simulink model "SF015A_WhlImbRejctn"  (R2013b)
settings: Solver=FixedStepDiscrete  SolverMode=SingleTasking  StartTime=0.0  StopTime=1  FixedStep=0.002  RelTol=1e-3
values from neighbouring files (symbols this model uses):
  ACTIVBANDMAX_ULS_U32 = DataDict.Constant    [SF015A_WhlImbRejctn_DataDict.m]
  ADAPVFILMAX_ULS_F32 = DataDict.Constant    [SF015A_WhlImbRejctn_DataDict.m]
  ARCHGLBPRM_180OVERPI_ULS_F32 = DataDict.Constant    [SF015A_WhlImbRejctn_DataDict.m]
  ARCHGLBPRM_2MILLISEC_SEC_F32 = DataDict.Constant    [SF015A_WhlImbRejctn_DataDict.m]
  ARCHGLBPRM_2PI_ULS_F32 = DataDict.Constant    [SF015A_WhlImbRejctn_DataDict.m]
  ARCHGLBPRM_FLOATZEROTHD_ULS_F32 = DataDict.Constant    [SF015A_WhlImbRejctn_DataDict.m]
  ARCHGLBPRM_PI_ULS_F32 = DataDict.Constant    [SF015A_WhlImbRejctn_DataDict.m]
  ARCHGLBPRM_PIOVER180_ULS_F32 = DataDict.Constant    [SF015A_WhlImbRejctn_DataDict.m]
  ARCHGLBPRM_PIOVER2_ULS_F32 = DataDict.Constant    [SF015A_WhlImbRejctn_DataDict.m]
  CALMINSPERCOUNT_ULS_F32 = DataDict.Constant    [SF015A_WhlImbRejctn_DataDict.m]
  DURATIONDISABLE_CNT_U16 = DataDict.Constant    [SF015A_WhlImbRejctn_DataDict.m]
  FILTWHLSPDMAX_MOTRADPERSEC_F32 = DataDict.Constant    [SF015A_WhlImbRejctn_DataDict.m]
  MICROSECTOMILLISEC_ULS_F32 = DataDict.Constant    [SF015A_WhlImbRejctn_DataDict.m]
  MINSTOMILLISEC_ULS_F32 = DataDict.Constant    [SF015A_WhlImbRejctn_DataDict.m]
  NINETY_ULS_F32 = DataDict.Constant    [SF015A_WhlImbRejctn_DataDict.m]
  NODEBSTEP_CNT_U16 = DataDict.Constant    [SF015A_WhlImbRejctn_DataDict.m]
  NROFDLY_CNT_U08 = DataDict.Constant    [SF015A_WhlImbRejctn_DataDict.m]
  ONEHALF_ULS_F32 = DataDict.Constant    [SF015A_WhlImbRejctn_DataDict.m]
  ONEHUNDRED_ULS_F32 = DataDict.Constant    [SF015A_WhlImbRejctn_DataDict.m]
  ONEOVRTHREE_ULS_F32 = DataDict.Constant    [SF015A_WhlImbRejctn_DataDict.m]
  ONEOVRTWENTY_ULS_F32 = DataDict.Constant    [SF015A_WhlImbRejctn_DataDict.m]
  ONETHOUSAND_ULS_F32 = DataDict.Constant    [SF015A_WhlImbRejctn_DataDict.m]
  PEAKMAX_ULS_F32 = DataDict.Constant    [SF015A_WhlImbRejctn_DataDict.m]
  PEAKMIN_ULS_F32 = DataDict.Constant    [SF015A_WhlImbRejctn_DataDict.m]
  PHAADJMAX_ULS_F32 = DataDict.Constant    [SF015A_WhlImbRejctn_DataDict.m]
  PITIMESSAMPLETIME_ULS_F32 = DataDict.Constant    [SF015A_WhlImbRejctn_DataDict.m]
  STOREDMINSPERCOUNT_ULS_F32 = DataDict.Constant    [SF015A_WhlImbRejctn_DataDict.m]
  TWO_ULS_F32 = DataDict.Constant    [SF015A_WhlImbRejctn_DataDict.m]
  TWOOVRTHREE_ULS_F32 = DataDict.Constant    [SF015A_WhlImbRejctn_DataDict.m]
  WhlImbRejctnAdpvFac = DataDict.Calibration    [SF015A_WhlImbRejctn_DataDict.m]
  WhlImbRejctnAutScaEna = DataDict.Calibration    [SF015A_WhlImbRejctn_DataDict.m]
  WhlImbRejctnAutScaTar = DataDict.Calibration    [SF015A_WhlImbRejctn_DataDict.m]
  WhlImbRejctnCurrMgnSlewPerLoop = DataDict.Calibration    [SF015A_WhlImbRejctn_DataDict.m]
  WhlImbRejctnDcTrendFltRcvryDly = DataDict.Calibration    [SF015A_WhlImbRejctn_DataDict.m]
  WhlImbRejctnDcTrendFltRcvryNegStep = DataDict.Calibration    [SF015A_WhlImbRejctn_DataDict.m]
  WhlImbRejctnDcTrendFltRcvryPosStep = DataDict.Calibration    [SF015A_WhlImbRejctn_DataDict.m]
  WhlImbRejctnDcTrendFltRcvryThd = DataDict.Calibration    [SF015A_WhlImbRejctn_DataDict.m]
  WhlImbRejctnDcTrendTh2Tq = DataDict.Calibration    [SF015A_WhlImbRejctn_DataDict.m]
  WhlImbRejctnDcTrendThTq = DataDict.Calibration    [SF015A_WhlImbRejctn_DataDict.m]
  WhlImbRejctnDcTrendTi2Sec = DataDict.Calibration    [SF015A_WhlImbRejctn_DataDict.m]
  WhlImbRejctnDcTrendTiSec = DataDict.Calibration    [SF015A_WhlImbRejctn_DataDict.m]
  WhlImbRejctnEnaSlewPerLoop = DataDict.Calibration    [SF015A_WhlImbRejctn_DataDict.m]
  WhlImbRejctnFctEna = DataDict.Calibration    [SF015A_WhlImbRejctn_DataDict.m]
  WhlImbRejctnFrqDiagcAmpThd = DataDict.Calibration    [SF015A_WhlImbRejctn_DataDict.m]
  WhlImbRejctnFrqDiagcEna = DataDict.Calibration    [SF015A_WhlImbRejctn_DataDict.m]
  WhlImbRejctnFrqDiagcFltRcvryDly = DataDict.Calibration    [SF015A_WhlImbRejctn_DataDict.m]
  WhlImbRejctnFrqDiagcFltRcvryNegStep = DataDict.Calibration    [SF015A_WhlImbRejctn_DataDict.m]
  WhlImbRejctnFrqDiagcFltRcvryPosStep = DataDict.Calibration    [SF015A_WhlImbRejctn_DataDict.m]
  WhlImbRejctnFrqDiagcFltRcvryThd = DataDict.Calibration    [SF015A_WhlImbRejctn_DataDict.m]
  WhlImbRejctnFrqDiagcThd = DataDict.Calibration    [SF015A_WhlImbRejctn_DataDict.m]
  WhlImbRejctnFrqDiagcTout = DataDict.Calibration    [SF015A_WhlImbRejctn_DataDict.m]
  WhlImbRejctnFrqDiagcUgrPoleMgn = DataDict.Calibration    [SF015A_WhlImbRejctn_DataDict.m]
  WhlImbRejctnFrqScaTblX = DataDict.Calibration    [SF015A_WhlImbRejctn_DataDict.m]
  WhlImbRejctnMaxDurn = DataDict.Calibration    [SF015A_WhlImbRejctn_DataDict.m]
  WhlImbRejctnMaxMgn = DataDict.Calibration    [SF015A_WhlImbRejctn_DataDict.m]
  WhlImbRejctnMaxMgnFltNegStep = DataDict.Calibration    [SF015A_WhlImbRejctn_DataDict.m]
  WhlImbRejctnMaxMgnFltPosStep = DataDict.Calibration    [SF015A_WhlImbRejctn_DataDict.m]
  WhlImbRejctnMaxMgnFltRcvryDly = DataDict.Calibration    [SF015A_WhlImbRejctn_DataDict.m]
  WhlImbRejctnMaxMgnFltRcvryNegStep = DataDict.Calibration    [SF015A_WhlImbRejctn_DataDict.m]
  WhlImbRejctnMaxMgnFltRcvryPosStep = DataDict.Calibration    [SF015A_WhlImbRejctn_DataDict.m]
  WhlImbRejctnMaxMgnFltRcvryThd = DataDict.Calibration    [SF015A_WhlImbRejctn_DataDict.m]
  WhlImbRejctnMaxMgnFltThd = DataDict.Calibration    [SF015A_WhlImbRejctn_DataDict.m]
  WhlImbRejctnMgnEstimnDeltaSca = DataDict.Calibration    [SF015A_WhlImbRejctn_DataDict.m]
  WhlImbRejctnMgnEstimnDiThd = DataDict.Calibration    [SF015A_WhlImbRejctn_DataDict.m]
  WhlImbRejctnMgnEstimnEnaThd = DataDict.Calibration    [SF015A_WhlImbRejctn_DataDict.m]
  WhlImbRejctnMgnEstimnFrq = DataDict.Calibration    [SF015A_WhlImbRejctn_DataDict.m]
  WhlImbRejctnMgnEstimnFrqDelta = DataDict.Calibration    [SF015A_WhlImbRejctn_DataDict.m]
  WhlImbRejctnMgnEstimnLeak = DataDict.Calibration    [SF015A_WhlImbRejctn_DataDict.m]
  WhlImbRejctnRampDwnTi = DataDict.Calibration    [SF015A_WhlImbRejctn_DataDict.m]
  WhlImbRejctnScaCncl = DataDict.Calibration    [SF015A_WhlImbRejctn_DataDict.m]
  WhlImbRejctnUgrPoleMgn = DataDict.Calibration    [SF015A_WhlImbRejctn_DataDict.m]
  WhlImbRejctnVehSpdEna = DataDict.Calibration    [SF015A_WhlImbRejctn_DataDict.m]
  WhlImbRejctnWhlSpdCorrlnFltRcvryDly = DataDict.Calibration    [SF015A_WhlImbRejctn_DataDict.m]
  WhlImbRejctnWhlSpdCorrlnFltRcvryNegStep = DataDict.Calibration    [SF015A_WhlImbRejctn_DataDict.m]
  WhlImbRejctnWhlSpdCorrlnFltRcvryPosStep = DataDict.Calibration    [SF015A_WhlImbRejctn_DataDict.m]
  WhlImbRejctnWhlSpdCorrlnFltRcvryThd = DataDict.Calibration    [SF015A_WhlImbRejctn_DataDict.m]
  WhlImbRejctnWhlSpdCorrlnThd = DataDict.Calibration    [SF015A_WhlImbRejctn_DataDict.m]
  WhlImbRejctnWhlSpdCorrlnTi = DataDict.Calibration    [SF015A_WhlImbRejctn_DataDict.m]
  WIRCMDMAX_MOTNWTMTR_F32 = DataDict.Constant    [SF015A_WhlImbRejctn_DataDict.m]
  ZERO_ULS_F32 = DataDict.Constant    [SF015A_WhlImbRejctn_DataDict.m]
undefined symbols (not defined in the file or in its folder): Cntr, NtcNr1, NvmGetErrSts1, SigQlfr1, Sts, SysSt1
libraries: simulink x32, FixdToFloat x32, Fil x20, NxtrLim x15, NxtrNvM x12, NxtrAbslt x8, NxtrMath x7, NxtrMax x6, NxtrMin x4, FloatToFixd x2, LnrIntrpn x2, NxtrSign x1
(part 5 of 12)

== system SF015A_WhlImbRejctn/WhlImbRejctn/WhlImbRejctnPer2/Flt Recovery- DC Trend/Update Fault Status ==
  Structvar : Inport
  Status : Inport  Port=2
  Bus Assignment : BusAssignment  AssignedSignals=Cntr,Sts
  Bus Selector : BusSelector  OutputSignals=Cntr,Sts,Thd,NegStep,PosStep
  Compare To Zero : simulink/Logic and Bit Operations/Compare To Zero  relop=<=  OutDataTypeStr=boolean
  Constant : Constant  Value=0  OutDataTypeStr=single
  CopyRight2 : Subsystem  Description=|  mask(Copyright Information){none=on}
      | Copyright info block.                                               
      |                                                                     
      | Place copyright information at the top of every subsystem in design.
      mask prompts: none "No parameters"
      mask help: Place copyright information at the top of every subsystem in design.
      mask Display:
      | NxtrConf = 'Nexteer Confidential';
      | 
      | sys = bdroot; %handle for the current model ("system")
      | first = get_param(sys,'Created');
      | first = first(end-3:end);  %year is last four digits
      | 
      | last = get_param(sys,'LastModifiedDate');
      | if isempty(last)
      |     last = datestr(now,'yyyy');
      | else
      |     last = last(end-3:end);
      | end
      | 
      | if strcmp(first,last)
      |     fprintf('%s -- Copyright %s Nexteer',NxtrConf,first)
      | else
      |     fprintf('%s -- %s%s- %s Nexteer',NxtrConf,char(169),first,last)
      | end
  Enumerated Constant : simulink/Sources/Enumerated Constant  OutDataTypeStr=Enum: SigQlfr1  Value=SigQlfr1.SIGQLFR_FAILD  SampleTime=inf
  Enumerated Constant1 : simulink/Sources/Enumerated Constant  OutDataTypeStr=Enum: SigQlfr1  Value=SigQlfr1.SIGQLFR_PASSD  SampleTime=inf
  If : If  IfExpression=u1
  If1 : If  NumInputs=2  IfExpression=u1  ElseIfExpressions=u2  ShowElse=off
  Merge : Merge
  Relational Operator : RelationalOperator  OutDataTypeStr=boolean
  Terminator : Terminator
  Towards Failed : Subsystem  TreatAsAtomicUnit=on
  Towards Passed : Subsystem  TreatAsAtomicUnit=on
  Update to Failed : Subsystem  TreatAsAtomicUnit=on
  Update to Passed : Subsystem  TreatAsAtomicUnit=on
  counter : Merge
  Structvar_out : Outport
  wires:
  Structvar/1 -> Bus Assignment/1, Bus Selector/1
  Status/1 -> If/1
  If/1 -> Towards Failed/Action
  If/2 -> Towards Passed/Action
  [PosStep] -> Towards Failed/1(PosStep)
  [NegStep] -> Towards Passed/1(NegStep)
  Towards Failed/1(Out1) -> counter/1
  Towards Passed/1(Out1) -> counter/2
  [Cnt] -> Towards Failed/2(Cnt)
  [Thd] -> Towards Failed/3(Thd)
  Constant/1 -> Towards Passed/3(Thd)
  counter/1 -> [Cnt_update], Compare To Zero/1, Relational Operator/1
  Relational Operator/1 -> If1/1
  If1/1 -> Update to Failed/Action
  If1/2 -> Update to Passed/Action
  Compare To Zero/1 -> If1/2
  Enumerated Constant1/1 -> Update to Passed/1(In1)
  Update to Failed/1(Out1) -> Merge/1
  Update to Passed/1(Out1) -> Merge/2
  Enumerated Constant/1 -> Update to Failed/1(In1)
  Bus Assignment/1 -> Structvar_out/1
  Merge/1 -> [Sts_update]
  Bus Selector/1 -> [Cnt]  "<Cntr>"
  Bus Selector/3 -> [Thd]  "<Thd>"
  Bus Selector/4 -> [NegStep]  "<NegStep>"
  Bus Selector/5 -> [PosStep]  "<PosStep>"
  [Cnt_update] -> Bus Assignment/2
  [Sts_update] -> Bus Assignment/3
  [Cnt] -> Towards Passed/2(Cnt)
  [Thd] -> Relational Operator/2
  Bus Selector/2 -> Terminator/1  "<Sts>"

== system SF015A_WhlImbRejctn/WhlImbRejctn/WhlImbRejctnPer2/Flt Recovery- Freq Diag/CopyRight2 ==

== system SF015A_WhlImbRejctn/WhlImbRejctn/WhlImbRejctnPer2/Flt Recovery- Freq Diag/ElapsedTime1 ==
  FltStsTrue : Inport
  CopyRight2 : Subsystem  Description=|  mask(Copyright Information){none=on}
      | Copyright info block.                                               
      |                                                                     
      | Place copyright information at the top of every subsystem in design.
      mask prompts: none "No parameters"
      mask help: Place copyright information at the top of every subsystem in design.
      mask Display:
      | NxtrConf = 'Nexteer Confidential';
      | 
      | sys = bdroot; %handle for the current model ("system")
      | first = get_param(sys,'Created');
      | first = first(end-3:end);  %year is last four digits
      | 
      | last = get_param(sys,'LastModifiedDate');
      | if isempty(last)
      |     last = datestr(now,'yyyy');
      | else
      |     last = last(end-3:end);
      | end
      | 
      | if strcmp(first,last)
      |     fprintf('%s -- Copyright %s Nexteer',NxtrConf,first)
      | else
      |     fprintf('%s -- %s%s- %s Nexteer',NxtrConf,char(169),first,last)
      | end
  Data Store Read : DataStoreRead  Priority=1  DataStoreName=FrqDiagcLrngEnaPrev
      settings: AttributesFormatString="priority:  %<Priority>"
  Data Store Write : DataStoreWrite  Priority=2  DataStoreName=FrqDiagcLrngEnaPrev
      settings: AttributesFormatString="priority:  %<Priority>"
  If : If  NumInputs=2  IfExpression=u1  ElseIfExpressions=u2
  If not true elapsed time = 0 : Subsystem  TreatAsAtomicUnit=on
  "If true and last step is true calculate elapsed time " : Subsystem  TreatAsAtomicUnit=on
  "If true and last step not true elapsed time = 0 get reference time " : Subsystem  TreatAsAtomicUnit=on
  Logical Operator1 : Logic  Operator=NOT  AllPortsSameDT=off  OutDataTypeStr=boolean
  Logical Operator2 : Logic  Operator=NOT  AllPortsSameDT=off  OutDataTypeStr=boolean
  Merge : Merge  Inputs=3
  ElapsedTime : Outport
  wires:
  If/1 -> If not true elapsed time = 0/Action
  If/2 -> "If true and last step not true elapsed time = 0 get reference time "/Action
  If/3 -> "If true and last step is true calculate elapsed time "/Action
  If not true elapsed time = 0/1(SpanTi) -> Merge/1
  "If true and last step not true elapsed time = 0 get reference time "/1("SpanTi ") -> Merge/2
  "If true and last step is true calculate elapsed time "/1(SpanTi) -> Merge/3
  Merge/1 -> ElapsedTime/1
  FltStsTrue/1 -> Logical Operator2/1, Data Store Write/1
  Data Store Read/1 -> Logical Operator1/1
  Logical Operator2/1 -> If/1
  Logical Operator1/1 -> If/2

== system SF015A_WhlImbRejctn/WhlImbRejctn/WhlImbRejctnPer2/Flt Recovery- Freq Diag/Update Fault Status ==
  Structvar : Inport
  Status : Inport  Port=2
  Bus Assignment : BusAssignment  AssignedSignals=Cntr,Sts
  Bus Selector : BusSelector  OutputSignals=Cntr,Sts,Thd,NegStep,PosStep
  Compare To Zero : simulink/Logic and Bit Operations/Compare To Zero  relop=<=  OutDataTypeStr=boolean
  Constant : Constant  Value=0  OutDataTypeStr=single
  CopyRight2 : Subsystem  Description=|  mask(Copyright Information){none=on}
      | Copyright info block.                                               
      |                                                                     
      | Place copyright information at the top of every subsystem in design.
      mask prompts: none "No parameters"
      mask help: Place copyright information at the top of every subsystem in design.
      mask Display:
      | NxtrConf = 'Nexteer Confidential';
      | 
      | sys = bdroot; %handle for the current model ("system")
      | first = get_param(sys,'Created');
      | first = first(end-3:end);  %year is last four digits
      | 
      | last = get_param(sys,'LastModifiedDate');
      | if isempty(last)
      |     last = datestr(now,'yyyy');
      | else
      |     last = last(end-3:end);
      | end
      | 
      | if strcmp(first,last)
      |     fprintf('%s -- Copyright %s Nexteer',NxtrConf,first)
      | else
      |     fprintf('%s -- %s%s- %s Nexteer',NxtrConf,char(169),first,last)
      | end
  Enumerated Constant : simulink/Sources/Enumerated Constant  OutDataTypeStr=Enum: SigQlfr1  Value=SigQlfr1.SIGQLFR_FAILD  SampleTime=inf
  Enumerated Constant1 : simulink/Sources/Enumerated Constant  OutDataTypeStr=Enum: SigQlfr1  Value=SigQlfr1.SIGQLFR_PASSD  SampleTime=inf
  If : If  IfExpression=u1
  If1 : If  NumInputs=2  IfExpression=u1  ElseIfExpressions=u2  ShowElse=off
  Merge : Merge
  Relational Operator : RelationalOperator  OutDataTypeStr=boolean
  Terminator : Terminator
  Towards Failed : Subsystem  TreatAsAtomicUnit=on
  Towards Passed : Subsystem  TreatAsAtomicUnit=on
  Update to Failed : Subsystem  TreatAsAtomicUnit=on
  Update to Passed : Subsystem  TreatAsAtomicUnit=on
  counter : Merge
  Structvar_out : Outport
  wires:
  Structvar/1 -> Bus Assignment/1, Bus Selector/1
  Status/1 -> If/1
  If/1 -> Towards Failed/Action
  If/2 -> Towards Passed/Action
  [PosStep] -> Towards Failed/1(PosStep)
  [NegStep] -> Towards Passed/1(NegStep)
  Towards Failed/1(Out1) -> counter/1
  Towards Passed/1(Out1) -> counter/2
  [Cnt] -> Towards Failed/2(Cnt)
  [Thd] -> Towards Failed/3(Thd)
  Constant/1 -> Towards Passed/3(Thd)
  counter/1 -> [Cnt_update], Compare To Zero/1, Relational Operator/1
  Relational Operator/1 -> If1/1
  If1/1 -> Update to Failed/Action
  If1/2 -> Update to Passed/Action
  Compare To Zero/1 -> If1/2
  Enumerated Constant1/1 -> Update to Passed/1(In1)
  Update to Failed/1(Out1) -> Merge/1
  Update to Passed/1(Out1) -> Merge/2
  Enumerated Constant/1 -> Update to Failed/1(In1)
  Bus Assignment/1 -> Structvar_out/1
  Merge/1 -> [Sts_update]
  Bus Selector/1 -> [Cnt]  "<Cntr>"
  Bus Selector/3 -> [Thd]  "<Thd>"
  Bus Selector/4 -> [NegStep]  "<NegStep>"
  Bus Selector/5 -> [PosStep]  "<PosStep>"
  [Cnt_update] -> Bus Assignment/2
  [Sts_update] -> Bus Assignment/3
  [Cnt] -> Towards Passed/2(Cnt)
  [Thd] -> Relational Operator/2
  Bus Selector/2 -> Terminator/1  "<Sts>"

== system SF015A_WhlImbRejctn/WhlImbRejctn/WhlImbRejctnPer2/Flt Recovery- Max Mag/CopyRight2 ==

== system SF015A_WhlImbRejctn/WhlImbRejctn/WhlImbRejctnPer2/Flt Recovery- Max Mag/ElapsedTime1 ==
  FltStsTrue : Inport
  CopyRight2 : Subsystem  Description=|  mask(Copyright Information){none=on}
      | Copyright info block.                                               
      |                                                                     
      | Place copyright information at the top of every subsystem in design.
      mask prompts: none "No parameters"
      mask help: Place copyright information at the top of every subsystem in design.
      mask Display:
      | NxtrConf = 'Nexteer Confidential';
      | 
      | sys = bdroot; %handle for the current model ("system")
      | first = get_param(sys,'Created');
      | first = first(end-3:end);  %year is last four digits
      | 
      | last = get_param(sys,'LastModifiedDate');
      | if isempty(last)
      |     last = datestr(now,'yyyy');
      | else
      |     last = last(end-3:end);
      | end
      | 
      | if strcmp(first,last)
      |     fprintf('%s -- Copyright %s Nexteer',NxtrConf,first)
      | else
      |     fprintf('%s -- %s%s- %s Nexteer',NxtrConf,char(169),first,last)
      | end
  Data Store Read : DataStoreRead  Priority=1  DataStoreName=MaxMgnLrngEnaPrev
      settings: AttributesFormatString="priority:  %<Priority>"
  Data Store Write : DataStoreWrite  Priority=2  DataStoreName=MaxMgnLrngEnaPrev
      settings: AttributesFormatString="priority:  %<Priority>"
  If : If  NumInputs=2  IfExpression=u1  ElseIfExpressions=u2
  If not true elapsed time = 0 : Subsystem  TreatAsAtomicUnit=on
  "If true and last step is true calculate elapsed time " : Subsystem  TreatAsAtomicUnit=on
  "If true and last step not true elapsed time = 0 get reference time " : Subsystem  TreatAsAtomicUnit=on
  Logical Operator1 : Logic  Operator=NOT  AllPortsSameDT=off  OutDataTypeStr=boolean
  Logical Operator2 : Logic  Operator=NOT  AllPortsSameDT=off  OutDataTypeStr=boolean
  Merge : Merge  Inputs=3
  ElapsedTime : Outport
  wires:
  If/1 -> If not true elapsed time = 0/Action
  If/2 -> "If true and last step not true elapsed time = 0 get reference time "/Action
  If/3 -> "If true and last step is true calculate elapsed time "/Action
  If not true elapsed time = 0/1(SpanTi) -> Merge/1
  "If true and last step not true elapsed time = 0 get reference time "/1("SpanTi ") -> Merge/2
  "If true and last step is true calculate elapsed time "/1(SpanTi) -> Merge/3
  Merge/1 -> ElapsedTime/1
  FltStsTrue/1 -> Logical Operator2/1, Data Store Write/1
  Data Store Read/1 -> Logical Operator1/1
  Logical Operator2/1 -> If/1
  Logical Operator1/1 -> If/2

== system SF015A_WhlImbRejctn/WhlImbRejctn/WhlImbRejctnPer2/Flt Recovery- Max Mag/Update Fault Status ==
  Structvar : Inport
  Status : Inport  Port=2
  Bus Assignment : BusAssignment  AssignedSignals=Cntr,Sts
  Bus Selector : BusSelector  OutputSignals=Cntr,Sts,Thd,NegStep,PosStep
  Compare To Zero : simulink/Logic and Bit Operations/Compare To Zero  relop=<=  OutDataTypeStr=boolean
  Constant : Constant  Value=0  OutDataTypeStr=single
  CopyRight2 : Subsystem  Description=|  mask(Copyright Information){none=on}
      | Copyright info block.                                               
      |                                                                     
      | Place copyright information at the top of every subsystem in design.
      mask prompts: none "No parameters"
      mask help: Place copyright information at the top of every subsystem in design.
      mask Display:
      | NxtrConf = 'Nexteer Confidential';
      | 
      | sys = bdroot; %handle for the current model ("system")
      | first = get_param(sys,'Created');
      | first = first(end-3:end);  %year is last four digits
      | 
      | last = get_param(sys,'LastModifiedDate');
      | if isempty(last)
      |     last = datestr(now,'yyyy');
      | else
      |     last = last(end-3:end);
      | end
      | 
      | if strcmp(first,last)
      |     fprintf('%s -- Copyright %s Nexteer',NxtrConf,first)
      | else
      |     fprintf('%s -- %s%s- %s Nexteer',NxtrConf,char(169),first,last)
      | end
  Enumerated Constant : simulink/Sources/Enumerated Constant  OutDataTypeStr=Enum: SigQlfr1  Value=SigQlfr1.SIGQLFR_FAILD  SampleTime=inf
  Enumerated Constant1 : simulink/Sources/Enumerated Constant  OutDataTypeStr=Enum: SigQlfr1  Value=SigQlfr1.SIGQLFR_PASSD  SampleTime=inf
  If : If  IfExpression=u1
  If1 : If  NumInputs=2  IfExpression=u1  ElseIfExpressions=u2  ShowElse=off
  Merge : Merge
  Relational Operator : RelationalOperator  OutDataTypeStr=boolean
  Terminator : Terminator
  Towards Failed : Subsystem  TreatAsAtomicUnit=on
  Towards Passed : Subsystem  TreatAsAtomicUnit=on
  Update to Failed : Subsystem  TreatAsAtomicUnit=on
  Update to Passed : Subsystem  TreatAsAtomicUnit=on
  counter : Merge
  Structvar_out : Outport
  wires:
  Structvar/1 -> Bus Assignment/1, Bus Selector/1
  Status/1 -> If/1
  If/1 -> Towards Failed/Action
  If/2 -> Towards Passed/Action
  [PosStep] -> Towards Failed/1(PosStep)
  [NegStep] -> Towards Passed/1(NegStep)
  Towards Failed/1(Out1) -> counter/1
  Towards Passed/1(Out1) -> counter/2
  [Cnt] -> Towards Failed/2(Cnt)
  [Thd] -> Towards Failed/3(Thd)
  Constant/1 -> Towards Passed/3(Thd)
  counter/1 -> [Cnt_update], Compare To Zero/1, Relational Operator/1
  Relational Operator/1 -> If1/1
  If1/1 -> Update to Failed/Action
  If1/2 -> Update to Passed/Action
  Compare To Zero/1 -> If1/2
  Enumerated Constant1/1 -> Update to Passed/1(In1)
  Update to Failed/1(Out1) -> Merge/1
  Update to Passed/1(Out1) -> Merge/2
  Enumerated Constant/1 -> Update to Failed/1(In1)
  Bus Assignment/1 -> Structvar_out/1
  Merge/1 -> [Sts_update]
  Bus Selector/1 -> [Cnt]  "<Cntr>"
  Bus Selector/3 -> [Thd]  "<Thd>"
  Bus Selector/4 -> [NegStep]  "<NegStep>"
  Bus Selector/5 -> [PosStep]  "<PosStep>"
  [Cnt_update] -> Bus Assignment/2
  [Sts_update] -> Bus Assignment/3
  [Cnt] -> Towards Passed/2(Cnt)
  [Thd] -> Relational Operator/2
  Bus Selector/2 -> Terminator/1  "<Sts>"

== system SF015A_WhlImbRejctn/WhlImbRejctn/WhlImbRejctnPer2/Flt Recovery- WhlSpdCorr Diag/CopyRight2 ==

== system SF015A_WhlImbRejctn/WhlImbRejctn/WhlImbRejctnPer2/Flt Recovery- WhlSpdCorr Diag/ElapsedTime1 ==
  FltStsTrue : Inport
  CopyRight2 : Subsystem  Description=|  mask(Copyright Information){none=on}
      | Copyright info block.                                               
      |                                                                     
      | Place copyright information at the top of every subsystem in design.
      mask prompts: none "No parameters"
      mask help: Place copyright information at the top of every subsystem in design.
      mask Display:
      | NxtrConf = 'Nexteer Confidential';
      | 
      | sys = bdroot; %handle for the current model ("system")
      | first = get_param(sys,'Created');
      | first = first(end-3:end);  %year is last four digits
      | 
      | last = get_param(sys,'LastModifiedDate');
      | if isempty(last)
      |     last = datestr(now,'yyyy');
      | else
      |     last = last(end-3:end);
      | end
      | 
      | if strcmp(first,last)
      |     fprintf('%s -- Copyright %s Nexteer',NxtrConf,first)
      | else
      |     fprintf('%s -- %s%s- %s Nexteer',NxtrConf,char(169),first,last)
      | end
  Data Store Read : DataStoreRead  Priority=1  DataStoreName=WhlSpdCorrlnDiagcLrngEnaPrev
      settings: AttributesFormatString="priority:  %<Priority>"
  Data Store Write : DataStoreWrite  Priority=2  DataStoreName=WhlSpdCorrlnDiagcLrngEnaPrev
      settings: AttributesFormatString="priority:  %<Priority>"
  If : If  NumInputs=2  IfExpression=u1  ElseIfExpressions=u2
  If not true elapsed time = 0 : Subsystem  TreatAsAtomicUnit=on
  "If true and last step is true calculate elapsed time " : Subsystem  TreatAsAtomicUnit=on
  "If true and last step not true elapsed time = 0 get reference time " : Subsystem  TreatAsAtomicUnit=on
  Logical Operator1 : Logic  Operator=NOT  AllPortsSameDT=off  OutDataTypeStr=boolean
  Logical Operator2 : Logic  Operator=NOT  AllPortsSameDT=off  OutDataTypeStr=boolean
  Merge : Merge  Inputs=3
  ElapsedTime : Outport
  wires:
  If/1 -> If not true elapsed time = 0/Action
  If/2 -> "If true and last step not true elapsed time = 0 get reference time "/Action
  If/3 -> "If true and last step is true calculate elapsed time "/Action
  If not true elapsed time = 0/1(SpanTi) -> Merge/1
  "If true and last step not true elapsed time = 0 get reference time "/1("SpanTi ") -> Merge/2
  "If true and last step is true calculate elapsed time "/1(SpanTi) -> Merge/3
  Merge/1 -> ElapsedTime/1
  FltStsTrue/1 -> Logical Operator2/1, Data Store Write/1
  Data Store Read/1 -> Logical Operator1/1
  Logical Operator2/1 -> If/1
  Logical Operator1/1 -> If/2

== system SF015A_WhlImbRejctn/WhlImbRejctn/WhlImbRejctnPer2/Flt Recovery- WhlSpdCorr Diag/Update Fault Status ==
  Structvar : Inport
  Status : Inport  Port=2
  Bus Assignment : BusAssignment  AssignedSignals=Cntr,Sts
  Bus Selector : BusSelector  OutputSignals=Cntr,Sts,Thd,NegStep,PosStep
  Compare To Zero : simulink/Logic and Bit Operations/Compare To Zero  relop=<=  OutDataTypeStr=boolean
  Constant : Constant  Value=0  OutDataTypeStr=single
  CopyRight2 : Subsystem  Description=|  mask(Copyright Information){none=on}
      | Copyright info block.                                               
      |                                                                     
      | Place copyright information at the top of every subsystem in design.
      mask prompts: none "No parameters"
      mask help: Place copyright information at the top of every subsystem in design.
      mask Display:
      | NxtrConf = 'Nexteer Confidential';
      | 
      | sys = bdroot; %handle for the current model ("system")
      | first = get_param(sys,'Created');
      | first = first(end-3:end);  %year is last four digits
      | 
      | last = get_param(sys,'LastModifiedDate');
      | if isempty(last)
      |     last = datestr(now,'yyyy');
      | else
      |     last = last(end-3:end);
      | end
      | 
      | if strcmp(first,last)
      |     fprintf('%s -- Copyright %s Nexteer',NxtrConf,first)
      | else
      |     fprintf('%s -- %s%s- %s Nexteer',NxtrConf,char(169),first,last)
      | end
  Enumerated Constant : simulink/Sources/Enumerated Constant  OutDataTypeStr=Enum: SigQlfr1  Value=SigQlfr1.SIGQLFR_FAILD  SampleTime=inf
  Enumerated Constant1 : simulink/Sources/Enumerated Constant  OutDataTypeStr=Enum: SigQlfr1  Value=SigQlfr1.SIGQLFR_PASSD  SampleTime=inf
  If : If  IfExpression=u1
  If1 : If  NumInputs=2  IfExpression=u1  ElseIfExpressions=u2  ShowElse=off
  Merge : Merge
  Relational Operator : RelationalOperator  OutDataTypeStr=boolean
  Terminator : Terminator
  Towards Failed : Subsystem  TreatAsAtomicUnit=on
  Towards Passed : Subsystem  TreatAsAtomicUnit=on
  Update to Failed : Subsystem  TreatAsAtomicUnit=on
  Update to Passed : Subsystem  TreatAsAtomicUnit=on
  counter : Merge
  Structvar_out : Outport
  wires:
  Structvar/1 -> Bus Assignment/1, Bus Selector/1
  Status/1 -> If/1
  If/1 -> Towards Failed/Action
  If/2 -> Towards Passed/Action
  [PosStep] -> Towards Failed/1(PosStep)
  [NegStep] -> Towards Passed/1(NegStep)
  Towards Failed/1(Out1) -> counter/1
  Towards Passed/1(Out1) -> counter/2
  [Cnt] -> Towards Failed/2(Cnt)
  [Thd] -> Towards Failed/3(Thd)
  Constant/1 -> Towards Passed/3(Thd)
  counter/1 -> [Cnt_update], Compare To Zero/1, Relational Operator/1
  Relational Operator/1 -> If1/1
  If1/1 -> Update to Failed/Action
  If1/2 -> Update to Passed/Action
  Compare To Zero/1 -> If1/2
  Enumerated Constant1/1 -> Update to Passed/1(In1)
  Update to Failed/1(Out1) -> Merge/1
  Update to Passed/1(Out1) -> Merge/2
  Enumerated Constant/1 -> Update to Failed/1(In1)
  Bus Assignment/1 -> Structvar_out/1
  Merge/1 -> [Sts_update]
  Bus Selector/1 -> [Cnt]  "<Cntr>"
  Bus Selector/3 -> [Thd]  "<Thd>"
  Bus Selector/4 -> [NegStep]  "<NegStep>"
  Bus Selector/5 -> [PosStep]  "<PosStep>"
  [Cnt_update] -> Bus Assignment/2
  [Sts_update] -> Bus Assignment/3
  [Cnt] -> Towards Passed/2(Cnt)
  [Thd] -> Relational Operator/2
  Bus Selector/2 -> Terminator/1  "<Sts>"

== system SF015A_WhlImbRejctn/WhlImbRejctn/WhlImbRejctnPer2/WIR Low Speed Diagnostics/CopyRight2 ==

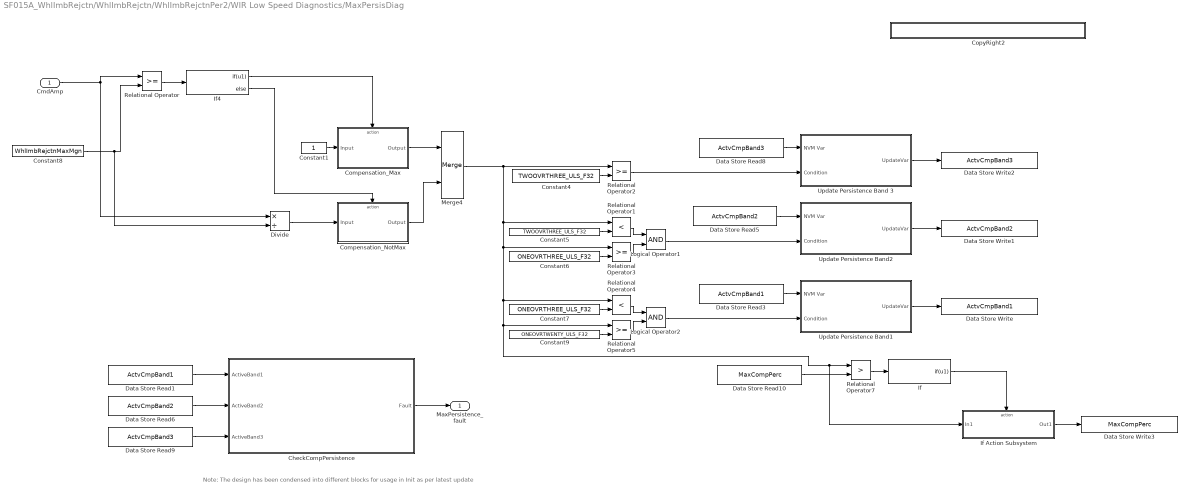
== system SF015A_WhlImbRejctn/WhlImbRejctn/WhlImbRejctnPer2/WIR Low Speed Diagnostics/MaxPersisDiag ==
  note: Note: The design has been condensed into different blocks for usage in Init as per latest update
  CmdAmp : Inport
  CheckCompPersistence : Subsystem
  Compensation_Max : Subsystem  RequirementInfo={} %GIDa_1bfe11f8_96f1_4e8d_9095_de3761426c03  TreatAsAtomicUnit=on
  Compensation_NotMax : Subsystem  RequirementInfo={} %GIDa_7b4c2964_e6f7_461b_b06a_d505129df27a  TreatAsAtomicUnit=on
  Constant1 : Constant  OutDataTypeStr=single
  Constant4 : Constant  Value=TWOOVRTHREE_ULS_F32
  Constant5 : Constant  Value=TWOOVRTHREE_ULS_F32
  Constant6 : Constant  Value=ONEOVRTHREE_ULS_F32
  Constant7 : Constant  Value=ONEOVRTHREE_ULS_F32
  Constant8 : Constant  Value=WhlImbRejctnMaxMgn
  Constant9 : Constant  Value=ONEOVRTWENTY_ULS_F32
  CopyRight2 : Subsystem  Description=|  mask(Copyright Information){none=on}
      | Copyright info block.                                               
      |                                                                     
      | Place copyright information at the top of every subsystem in design.
      mask prompts: none "No parameters"
      mask help: Place copyright information at the top of every subsystem in design.
      mask Display:
      | NxtrConf = 'Nexteer Confidential';
      | 
      | sys = bdroot; %handle for the current model ("system")
      | first = get_param(sys,'Created');
      | first = first(end-3:end);  %year is last four digits
      | 
      | last = get_param(sys,'LastModifiedDate');
      | if isempty(last)
      |     last = datestr(now,'yyyy');
      | else
      |     last = last(end-3:end);
      | end
      | 
      | if strcmp(first,last)
      |     fprintf('%s -- Copyright %s Nexteer',NxtrConf,first)
      | else
      |     fprintf('%s -- %s%s- %s Nexteer',NxtrConf,char(169),first,last)
      | end
  Data Store Read1 : DataStoreRead  Priority=3  DataStoreName=ActvCmpBand1
      settings: AttributesFormatString=Priority=%<Priority>
  Data Store Read10 : DataStoreRead  DataStoreName=MaxCompPerc
  Data Store Read3 : DataStoreRead  Priority=1  DataStoreName=ActvCmpBand1
      settings: AttributesFormatString=Priority=%<Priority>
  Data Store Read5 : DataStoreRead  Priority=1  DataStoreName=ActvCmpBand2
      settings: AttributesFormatString=Priority=%<Priority>
  Data Store Read6 : DataStoreRead  Priority=3  DataStoreName=ActvCmpBand2
      settings: AttributesFormatString=Priority=%<Priority>
  Data Store Read8 : DataStoreRead  Priority=1  DataStoreName=ActvCmpBand3
  Data Store Read9 : DataStoreRead  Priority=3  DataStoreName=ActvCmpBand3
      settings: AttributesFormatString=Priority=%<Priority>
  Data Store Write : DataStoreWrite  Priority=2  DataStoreName=ActvCmpBand1
      settings: AttributesFormatString=Priority=%<Priority>
  Data Store Write1 : DataStoreWrite  Priority=2  DataStoreName=ActvCmpBand2
      settings: AttributesFormatString=Priority=%<Priority>
  Data Store Write2 : DataStoreWrite  Priority=2  DataStoreName=ActvCmpBand3
      settings: AttributesFormatString=Priority=%<Priority>
  Data Store Write3 : DataStoreWrite  DataStoreName=MaxCompPerc
  Divide : Product  Inputs=*/
  If : If  IfExpression=u1  ShowElse=off
  If Action Subsystem : Subsystem  TreatAsAtomicUnit=on
  If4 : If  IfExpression=u1
  Logical Operator1 : Logic  AllPortsSameDT=off  OutDataTypeStr=boolean
  Logical Operator2 : Logic  AllPortsSameDT=off  OutDataTypeStr=boolean
  Merge4 : Merge
  Relational Operator{,2..3,5} (4 alike) : RelationalOperator  OutDataTypeStr=boolean
  Relational Operator1 : RelationalOperator  Operator=<  OutDataTypeStr=boolean
  Relational Operator4 : RelationalOperator  Operator=<  OutDataTypeStr=boolean
  Relational Operator7 : RelationalOperator  Operator=>  OutDataTypeStr=boolean
  Update Persistence Band 3 : Subsystem
  Update Persistence Band1 : Subsystem
  Update Persistence Band2 : Subsystem
  MaxPersistence_fault : Outport
  wires:
  CmdAmp/1 -> Relational Operator/1, Divide/1
  Constant8/1 -> Divide/2, Relational Operator/2
  Merge4/1 -> If Action Subsystem/1(In1), Relational Operator7/1, Relational Operator5/1, Relational Operator4/1, Relational Operator3/1, Relational Operator1/1, Relational Operator2/1
  Constant6/1 -> Relational Operator3/2
  Constant4/1 -> Relational Operator2/2
  Constant5/1 -> Relational Operator1/2
  Constant9/1 -> Relational Operator5/2
  Constant7/1 -> Relational Operator4/2
  Relational Operator3/1 -> Logical Operator1/2
  Relational Operator1/1 -> Logical Operator1/1
  Relational Operator4/1 -> Logical Operator2/1
  Relational Operator5/1 -> Logical Operator2/2
  Logical Operator1/1 -> Update Persistence Band2/2(Condition)
  Relational Operator7/1 -> If/1
  Data Store Read10/1 -> Relational Operator7/2
  If/1 -> If Action Subsystem/Action
  If Action Subsystem/1(Out1) -> Data Store Write3/1
  Relational Operator/1 -> If4/1
  Compensation_Max/1(Output) -> Merge4/1
  If4/1 -> Compensation_Max/Action
  Constant1/1 -> Compensation_Max/1(Input)
  Compensation_NotMax/1(Output) -> Merge4/2
  If4/2 -> Compensation_NotMax/Action
  Divide/1 -> Compensation_NotMax/1(Input)
  Data Store Read8/1 -> Update Persistence Band 3/1(NVM Var)
  Update Persistence Band 3/1(UpdateVar) -> Data Store Write2/1
  Relational Operator2/1 -> Update Persistence Band 3/2(Condition)
  Data Store Read5/1 -> Update Persistence Band2/1(NVM Var)
  Update Persistence Band2/1(UpdateVar) -> Data Store Write1/1
  Logical Operator2/1 -> Update Persistence Band1/2(Condition)
  Data Store Read3/1 -> Update Persistence Band1/1(NVM Var)
  Update Persistence Band1/1(UpdateVar) -> Data Store Write/1
  Data Store Read1/1 -> CheckCompPersistence/1(ActiveBand1)
  Data Store Read6/1 -> CheckCompPersistence/2(ActiveBand2)
  Data Store Read9/1 -> CheckCompPersistence/3(ActiveBand3)
  CheckCompPersistence/1(Fault) -> MaxPersistence_fault/1

== system SF015A_WhlImbRejctn/WhlImbRejctn/WhlImbRejctnInit1/Check NVM Data/CheckCompPersistence/CopyRight2 ==

== system SF015A_WhlImbRejctn/WhlImbRejctn/WhlImbRejctnInit1/Check NVM Data/CheckCompPersistence/NoFault ==
  Input : Inport
  Action Port : ActionPort  ActionType=else
  CopyRight2 : Subsystem  Description=|  mask(Copyright Information){none=on}
      | Copyright info block.                                               
      |                                                                     
      | Place copyright information at the top of every subsystem in design.
      mask prompts: none "No parameters"
      mask help: Place copyright information at the top of every subsystem in design.
      mask Display:
      | NxtrConf = 'Nexteer Confidential';
      | 
      | sys = bdroot; %handle for the current model ("system")
      | first = get_param(sys,'Created');
      | if(isempty(first))
      |     first = datestr(now,'yyyy');
      | else
      |     first = first(end-3:end);  %year is last four digits
      | end
      | 
      | last = get_param(sys,'LastModifiedDate');
      | if isempty(last)
      |     last = datestr(now,'yyyy');
      | else
      |     last = last(end-3:end);
      | end
      | 
      | if strcmp(first,last)
      |     fprintf('%s -- Copyright %s Nexteer',NxtrConf,first)
      | else
      |     fprintf('%s -- %s%s- %s Nexteer',NxtrConf,char(169),first,last)
      | end
  Output : Outport
  wires:
  Input/1 -> Output/1

== system SF015A_WhlImbRejctn/WhlImbRejctn/WhlImbRejctnInit1/Check NVM Data/CheckCompPersistence/Subsystem ==
  Band : Inport
  Band2 : Inport  Port=2
  Band3 : Inport  Port=3
  Action Port : ActionPort  ActionType=then
  Constant10 : Constant  Value=TWOOVRTHREE_ULS_F32
  Constant11 : Constant  Value=ONEOVRTHREE_ULS_F32
  Constant12 : Constant  Value=WhlImbRejctnMaxDurn
  Constant15 : Constant  Value=0  OutDataTypeStr=boolean
  Constant16 : Constant  OutDataTypeStr=boolean
  Constant17 : Constant  Value=STOREDMINSPERCOUNT_ULS_F32
  Constant2 : Constant  Value=CALMINSPERCOUNT_ULS_F32
  CopyRight1 : Subsystem  Description=|  mask(Copyright Information){none=on}
      | Copyright info block.                                               
      |                                                                     
      | Place copyright information at the top of every subsystem in design.
      mask prompts: none "No parameters"
      mask help: Place copyright information at the top of every subsystem in design.
      mask Display:
      | NxtrConf = 'Nexteer Confidential';
      | 
      | sys = bdroot; %handle for the current model ("system")
      | first = get_param(sys,'Created');
      | first = first(end-3:end);  %year is last four digits
      | 
      | last = get_param(sys,'LastModifiedDate');
      | if isempty(last)
      |     last = datestr(now,'yyyy');
      | else
      |     last = last(end-3:end);
      | end
      | 
      | if strcmp(first,last)
      |     fprintf('%s -- Copyright %s Nexteer',NxtrConf,first)
      | else
      |     fprintf('%s -- %s%s- %s Nexteer',NxtrConf,char(169),first,last)
      | end
  Data Type Conversion : DataTypeConversion  OutDataTypeStr=boolean
  Data Type Conversion1 : DataTypeConversion  OutDataTypeStr=boolean
  FixdToFloat_f32_u1 : FixdToFloat/FixdToFloat_f32_u32  Param1=0
  FixdToFloat_f32_u16 : FixdToFloat/FixdToFloat_f32_u16  Param1=0
  FixdToFloat_f32_u2 : FixdToFloat/FixdToFloat_f32_u32  Param1=0
  FixdToFloat_f32_u32 : FixdToFloat/FixdToFloat_f32_u32  Param1=0
  FreqDiagFault : Subsystem  RequirementInfo={} %GIDa_212db42b_1f35_4015_b5bf_9bd3bcd3665a  TreatAsAtomicUnit=on
  If5 : If  RequirementInfo={} %GIDa_d54da65b_dc62_4224_8642_661d9ee3c040  IfExpression=u1
  Merge5 : Merge
  NoFault : Subsystem  RequirementInfo={} %GIDa_c3beeaa0_bcda_4c66_a9c8_2ab73aa20fa7  TreatAsAtomicUnit=on
  Product : Product
  Product1 : Product
  Product2 : Product  RndMeth=Zero
  Product3 : Product  RndMeth=Zero
  Relational Operator6 : RelationalOperator  Operator=>  OutDataTypeStr=boolean
  Sum : Sum  Inputs=|+++
  Fault : Outport
  wires:
  Merge5/1 -> Fault/1
  Constant10/1 -> Product2/2
  Constant11/1 -> Product3/2
  Band3/1 -> FixdToFloat_f32_u2/1
  Band2/1 -> FixdToFloat_f32_u1/1
  Product3/1 -> Sum/3
  Product2/1 -> Sum/2
  Band/1 -> FixdToFloat_f32_u32/1
  Constant12/1 -> FixdToFloat_f32_u16/1
  Relational Operator6/1 -> If5/1
  If5/1 -> FreqDiagFault/Action
  If5/2 -> NoFault/Action
  FreqDiagFault/1(Output) -> Merge5/1
  NoFault/1(Output) -> Merge5/2
  Constant16/1 -> Data Type Conversion/1
  Constant15/1 -> Data Type Conversion1/1
  FixdToFloat_f32_u1/1 -> Product2/1
  FixdToFloat_f32_u2/1 -> Product3/1
  FixdToFloat_f32_u16/1 -> Product/1
  Data Type Conversion/1 -> FreqDiagFault/1(Input)
  Data Type Conversion1/1 -> NoFault/1(Input)
  FixdToFloat_f32_u32/1 -> Sum/1
  Constant17/1 -> Product1/2
  Product/1 -> Relational Operator6/2
  Product1/1 -> Relational Operator6/1
  Sum/1 -> Product1/1
  Constant2/1 -> Product/2

== system SF015A_WhlImbRejctn/WhlImbRejctn/WhlImbRejctnInit1/Check NVM Data/NvmNotVal/CopyRight2 ==

== system SF015A_WhlImbRejctn/WhlImbRejctn/WhlImbRejctnInit1/Check NVM Data/ResetNVM/CopyRight2 ==

== system SF015A_WhlImbRejctn/WhlImbRejctn/WhlImbRejctnInit1/Check NVM Data/ResetNVM1/CopyRight2 ==

== system SF015A_WhlImbRejctn/WhlImbRejctn/WhlImbRejctnPer1/Active Rejection Command /Phase Adjust - Floating Point/Calc Filter Coefficients ==
  phase : Inport
  freq : Inport  Port=2
  CalcCoeff : Subsystem
  CalcZeroPole : Subsystem
  z_m : Outport
  p_k : Outport  Port=2
  b_0 : Outport  Port=3
  1/Mag : Outport  Port=4
  wires:
  CalcZeroPole/4(1/Mag at freq) -> 1/Mag/1
  freq/1 -> CalcZeroPole/2(freq)
  CalcCoeff/3(b_0) -> b_0/1
  CalcCoeff/2(p_k) -> p_k/1
  phase/1 -> CalcZeroPole/1(phase)
  CalcCoeff/1(z_m) -> z_m/1
  CalcZeroPole/3(CompGain) -> CalcCoeff/3(gain)
  CalcZeroPole/2(pole) -> CalcCoeff/2(pole)
  CalcZeroPole/1(zero) -> CalcCoeff/1(zero)

== system SF015A_WhlImbRejctn/WhlImbRejctn/WhlImbRejctnPer1/Active Rejection Command /Phase Adjust - Floating Point/Filter 1 ==
  In1 : Inport
  z_m : Inport  Port=2
  p_k : Inport  Port=3
  b_0 : Inport  Port=4
  1/Mag : Inport  Port=5
  Add : Sum  Inputs=+-
  Add1 : Sum
  Constant1 : Constant  Value=PHAADJMAX_ULS_F32
  Data Store Read : DataStoreRead  DataStoreName=PhaAdjFil1Coeff2
  Data Store Read1 : DataStoreRead  Priority=1  DataStoreName=PhaAdjFil1Coeff1
      settings: AttributesFormatString=%<Priority 1>
  Data Store Write : DataStoreWrite  DataStoreName=PhaAdjFil1Coeff2
  Data Store Write1 : DataStoreWrite  Priority=2  DataStoreName=PhaAdjFil1Coeff1
      settings: AttributesFormatString=%<Priority 2>
  LimDyn_f32 : NxtrLim/LimDyn_f32
  Product : Product  RndMeth=Zero
  Product1 : Product  RndMeth=Zero
  Product2 : Product  RndMeth=Zero
  Product3 : Product  Inputs=**  RndMeth=Zero
  Unary Minus : UnaryMinus
  Out1 : Outport
  wires:
  b_0/1 -> [b_0_calc]
  [p_k_calc] -> Product2/2
  [z_m_calc] -> Product1/2
  p_k/1 -> [p_k_calc]
  z_m/1 -> [z_m_calc]
  In1/1 -> Data Store Write1/1, Add/1
  Product2/1 -> Add1/2
  Add1/1 -> Data Store Write/1, Product3/1
  Product/1 -> Add1/1
  [b_0_calc] -> Product/2
  Add/1 -> Product/1
  Product1/1 -> Add/2
  Data Store Read1/1 -> Product1/1  "x_n-1"
  1/Mag/1 -> Product3/2
  Data Store Read/1 -> Product2/1
  LimDyn_f32/1 -> Out1/1
  Constant1/1 -> Unary Minus/1, LimDyn_f32/3
  Unary Minus/1 -> LimDyn_f32/2
  Product3/1 -> LimDyn_f32/1

== system SF015A_WhlImbRejctn/WhlImbRejctn/WhlImbRejctnPer1/Active Rejection Command /Phase Adjust - Floating Point/Filter 2 ==
  In1 : Inport
  z_m : Inport  Port=2
  p_k : Inport  Port=3
  b_0 : Inport  Port=4
  1/Mag : Inport  Port=5
  Add : Sum  Inputs=+-
  Add1 : Sum
  Constant1 : Constant  Value=PHAADJMAX_ULS_F32
  Data Store Read : DataStoreRead  DataStoreName=PhaAdjFil2Coeff2
  Data Store Read1 : DataStoreRead  Priority=1  DataStoreName=PhaAdjFil2Coeff1
      settings: AttributesFormatString=%<Priority 1>
  Data Store Write : DataStoreWrite  DataStoreName=PhaAdjFil2Coeff2
  Data Store Write1 : DataStoreWrite  Priority=2  DataStoreName=PhaAdjFil2Coeff1
      settings: AttributesFormatString=%<Priority 2>
  LimDyn_f32 : NxtrLim/LimDyn_f32
  Product : Product  RndMeth=Zero
  Product1 : Product  RndMeth=Zero
  Product2 : Product  RndMeth=Zero
  Product3 : Product  Inputs=**  RndMeth=Zero
  Unary Minus : UnaryMinus
  Out1 : Outport
  wires:
  1/Mag/1 -> Product3/2
  Data Store Read1/1 -> Product1/1  "x_n-1"
  Product1/1 -> Add/2
  Add/1 -> Product/1
  [b_0_calc] -> Product/2
  Product/1 -> Add1/1
  Add1/1 -> Data Store Write/1, Product3/1
  Product2/1 -> Add1/2
  In1/1 -> Data Store Write1/1, Add/1
  z_m/1 -> [z_m_calc]
  p_k/1 -> [p_k_calc]
  [z_m_calc] -> Product1/2
  [p_k_calc] -> Product2/2
  b_0/1 -> [b_0_calc]
  Data Store Read/1 -> Product2/1
  Constant1/1 -> Unary Minus/1, LimDyn_f32/3
  Unary Minus/1 -> LimDyn_f32/2
  Product3/1 -> LimDyn_f32/1
  LimDyn_f32/1 -> Out1/1

== system SF015A_WhlImbRejctn/WhlImbRejctn/WhlImbRejctnPer1/Active Rejection Command /Phase Adjust - Floating Point/If Action Subsystem ==
  Pha_input : Inport
  PhaseInput : Inport  Port=2
  Action Port : ActionPort  ActionType=then
  Abslt_f32_f32 : NxtrAbslt/Abslt_f32_f32  SFunctionSpec=single y1 = Abslt_f32_f32(single u1)
      settings: AttributesFormatString=%<Name>
  Add : Sum  Inputs=-+
  Constant : Constant  Value=ARCHGLBPRM_PI_ULS_F32
  Constant1 : Constant  Value=ARCHGLBPRM_180OVERPI_ULS_F32
  Product : Product
  Product1 : Product
  Sign_s08_f32 : NxtrSign/Sign_s08_f32  SFunctionSpec=int8 y1 = Sign_s08_f32(single u1)
  Unary Minus : UnaryMinus
  Unary Minus1 : UnaryMinus
  Phase : Outport
  FinalPhaInput : Outport  Port=2
  wires:
  PhaseInput/1 -> Unary Minus/1
  Unary Minus/1 -> FinalPhaInput/1
  Sign_s08_f32/1 -> Unary Minus1/1
  Constant/1 -> Product/1
  Constant1/1 -> Product/2
  Product/1 -> Add/2
  Pha_input/1 -> Abslt_f32_f32/1, Sign_s08_f32/1
  Unary Minus1/1 -> Product1/1
  Add/1 -> Product1/2
  Product1/1 -> Phase/1
  Abslt_f32_f32/1 -> Add/1

== system SF015A_WhlImbRejctn/WhlImbRejctn/WhlImbRejctnPer1/Active Rejection Command /Phase Adjust - Floating Point/If Action Subsystem1 ==
  Pha_input : Inport
  PhaseInput : Inport  Port=2
  Action Port : ActionPort  ActionType=else
  Phase : Outport
  FinalPhaInput : Outport  Port=2
  wires:
  PhaseInput/1 -> FinalPhaInput/1
  Pha_input/1 -> Phase/1

== system SF015A_WhlImbRejctn/WhlImbRejctn/WhlImbRejctnPer1/Determine Enabled Amt/Calculate Enable1/Check_EnableDisableRange ==
  DistMagL : Inport
  DistMagR : Inport  Port=2
  DistMagEnadPrev : Inport  Port=3
  Check_for_disbale1 : Subsystem  RequirementInfo={} %GIDa_159aba51_987a_470b_b955_203c08afb92c  TreatAsAtomicUnit=on
  Check_for_disbale2 : Subsystem  RequirementInfo={} %GIDa_46258d0f_eb0e_4930_aedd_1583eb5dcf2e  TreatAsAtomicUnit=on
  Check_for_disbale3 : Subsystem  RequirementInfo={} %GIDa_a7256a8a_fc45_45b1_accf_cae14e85cdcb  TreatAsAtomicUnit=on
  Constant1 : Constant  OutDataTypeStr=boolean
  Constant12 : Constant  Value=WhlImbRejctnMgnEstimnEnaThd
  Constant15 : Constant  Value=0  OutDataTypeStr=boolean
  Constant2 : Constant  Value=0  OutDataTypeStr=boolean
  Constant5 : Constant  Value=WhlImbRejctnMgnEstimnDiThd
  CopyRight2 : Subsystem  Description=|  mask(Copyright Information){none=on}
      | Copyright info block.                                               
      |                                                                     
      | Place copyright information at the top of every subsystem in design.
      mask prompts: none "No parameters"
      mask help: Place copyright information at the top of every subsystem in design.
      mask Display:
      | NxtrConf = 'Nexteer Confidential';
      | 
      | sys = bdroot; %handle for the current model ("system")
      | first = get_param(sys,'Created');
      | first = first(end-3:end);  %year is last four digits
      | 
      | last = get_param(sys,'LastModifiedDate');
      | if isempty(last)
      |     last = datestr(now,'yyyy');
      | else
      |     last = last(end-3:end);
      | end
      | 
      | if strcmp(first,last)
      |     fprintf('%s -- Copyright %s Nexteer',NxtrConf,first)
      | else
      |     fprintf('%s -- %s%s- %s Nexteer',NxtrConf,char(169),first,last)
      | end
  Data Type Conversion1 : DataTypeConversion  OutDataTypeStr=boolean
  Data Type Conversion2 : DataTypeConversion  OutDataTypeStr=boolean
  Data Type Conversion3 : DataTypeConversion  OutDataTypeStr=boolean
  If10 : If  RequirementInfo={} %GIDa_918bc6d9_1c7e_43ab_b258_8fd3aaafebf7  NumInputs=2  IfExpression=u1  ElseIfExpressions=u2
  Logical Operator3 : Logic  AllPortsSameDT=off  OutDataTypeStr=boolean
  Logical Operator4 : Logic  Operator=OR  Inputs=3  AllPortsSameDT=off  OutDataTypeStr=boolean
  Merge6 : Merge  Inputs=3
  Relational Operator1 : RelationalOperator  Operator=>  OutDataTypeStr=boolean
  Relational Operator2 : RelationalOperator  Operator=<  OutDataTypeStr=boolean
  Relational Operator3 : RelationalOperator  Operator=>  OutDataTypeStr=boolean
  Relational Operator7 : RelationalOperator  Operator=<  OutDataTypeStr=boolean
  PrevEnabld : Outport
  wires:
  Logical Operator4/1 -> If10/2
  Merge6/1 -> PrevEnabld/1
  If10/3 -> Check_for_disbale3/Action
  Constant15/1 -> Data Type Conversion1/1
  Relational Operator2/1 -> Logical Operator3/1
  Constant5/1 -> Relational Operator2/2, Relational Operator7/2
  Relational Operator7/1 -> Logical Operator3/2
  If10/1 -> Check_for_disbale2/Action
  Logical Operator3/1 -> If10/1
  Data Type Conversion1/1 -> Check_for_disbale2/1(Input)
  DistMagR/1 -> [DistMagR]
  DistMagL/1 -> [DistMagL]
  DistMagEnadPrev/1 -> [DistMagEnadPrev]
  Check_for_disbale2/1(Output) -> Merge6/1
  [DistMagL] -> Relational Operator2/1
  [DistMagR] -> Relational Operator7/1
  [DistMagL] -> Relational Operator1/1
  [DistMagR] -> Relational Operator3/1
  Constant12/1 -> Relational Operator1/2, Relational Operator3/2
  Relational Operator1/1 -> Logical Operator4/1
  Relational Operator3/1 -> Logical Operator4/2
  [DistMagEnadPrev] -> Logical Operator4/3
  Constant1/1 -> Data Type Conversion2/1
  If10/2 -> Check_for_disbale1/Action
  Data Type Conversion2/1 -> Check_for_disbale1/1(Input)
  Check_for_disbale1/1(Output) -> Merge6/2
  Check_for_disbale3/1(Output) -> Merge6/3
  Constant2/1 -> Data Type Conversion3/1
  Data Type Conversion3/1 -> Check_for_disbale3/1(Input)
